simulink subsystem "CA_switch"  (R2025a)
settings: Solver=VariableStepAuto  StartTime=0.0  StopTime=10.0  RelTol=1e-3
settings Model: Creator=gurt1  LastModifiedBy=gurt1

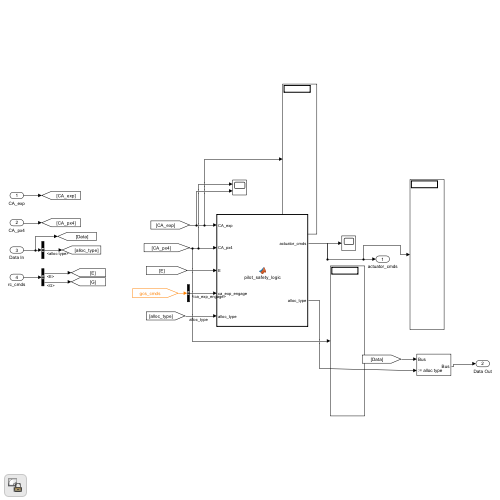
[thumbnail: Simulink's stored preview of the top-level diagram]
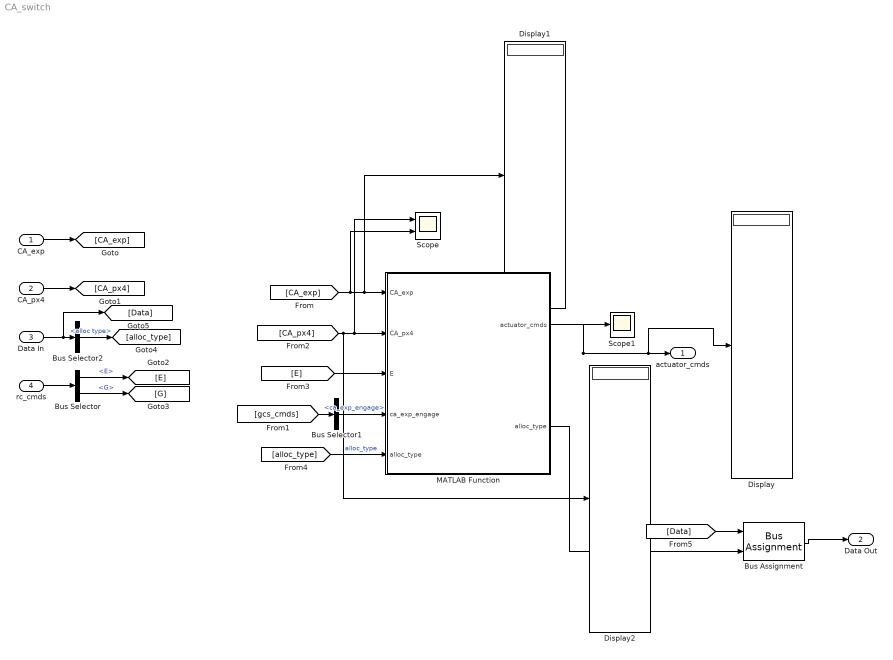
== system CA_switch ==
  CA_exp : Inport
  CA_px4 : Inport  Port=2
  Data In : Inport  Port=3
  rc_cmds : Inport  Port=4
  Bus Assignment : BusAssignment  AssignedSignals=alloc type
  Bus Selector : BusSelector  OutputSignals=switches.E,switches.G
  Bus Selector1 : BusSelector  OutputSignals=Fault.ca_exp_engage
  Bus Selector2 : BusSelector  OutputSignals=alloc type
  Display : Display
  Display1 : Display
  Display2 : Display
  MATLAB Function : MATLAB Function  TreatAsAtomicUnit=on
  Scope : Scope  NumInputPorts=2
      settings: ActiveDisplayYMinimum=-1.0204996857047082  ActiveDisplayYMaximum=2.21338885396719  DataLoggingVariableName=ScopeData7
  Scope1 : Scope
      settings: ActiveDisplayYMinimum=-1.3775  ActiveDisplayYMaximum=2.3975  DataLoggingVariableName=ScopeData9
  actuator_cmds : Outport
  Data Out : Outport  Port=2
  wires:
  CA_exp/1 -> [CA_exp]
  CA_px4/1 -> [CA_px4]
  rc_cmds/1 -> Bus Selector/1
  Bus Selector/1 -> [E]  "<E>"
  Bus Selector/2 -> [G]  "<G>"
  [gcs_cmds] -> Bus Selector1/1
  [CA_exp] -> MATLAB Function/1(CA_exp), Display1/1, Scope/2
  [CA_px4] -> Display2/1, MATLAB Function/2(CA_px4), Scope/1
  [E] -> MATLAB Function/3(E)
  Bus Selector1/1 -> MATLAB Function/4(ca_exp_engage)  "<ca_exp_engage>"
  MATLAB Function/1(actuator_cmds) -> actuator_cmds/1, Display/1, Scope1/1
  Data In/1 -> Bus Selector2/1, [Data]
  Bus Selector2/1 -> [alloc_type]  "<alloc type>"
  [alloc_type] -> MATLAB Function/5("alloc_type ")  "alloc_type"
  [Data] -> Bus Assignment/1
  Bus Assignment/1 -> Data Out/1
  MATLAB Function/2(alloc_type) -> Bus Assignment/2

== matlab function CA_switch/MATLAB Function ==
  data: CA_exp input; actuator_cmds output; CA_px4 input; E input; ca_exp_engage input; alloc_type input; alloc_type output
function [actuator_cmds,alloc_type] = pilot_safety_logic(CA_exp, CA_px4, E, ca_exp_engage, alloc_type) 
%% PILOT SAFETY SWITCH LOGIC
% DESCRIPTION:
%   Pilot "oh shite" override logic for control allocation selection.
%   If E > 0, force PX4 allocation. If E == 0 and ca_exp_engage > 0,
%   use experimental allocation; otherwise default to PX4.
%
% INPUTS:
%   CA_exp         - Experimental control allocation command vector [m x 1]
%   CA_px4         - PX4 control allocation command vector [m x 1]
%   E              - Pilot override switch (scalar; 0 = allow GS, >0 = force PX4)
%   ca_exp_engage  - Ground-station engage flag for experimental CA (scalar)
%
% OUTPUTS:
%   actuator_cmds  - Selected actuator command vector [m x 1]
%
% WRITTEN BY:
%   Garrett D. Asper
%   Virginia Tech
%   Email: garrettasper@vt.edu
%
% HISTORY:
%   28-Aug-2025 - Created and debugged, GDA
%
% NOMENCLATURE:                                  UNITS:
%   Not Applicable                                  Not Applicable.

% Default/fallback: trust PX4 allocation
actuator_cmds = CA_px4;

% Use experimental allocation only when E == 0 and GS has engaged it
if (E == 0) && (ca_exp_engage > 0)
    actuator_cmds = CA_exp;
    alloc_type = alloc_type; % let the experimental mode through
else 
    actuator_cmds = CA_px4;
    alloc_type = 0;          % override the experimental mode
end

end
